simulink model "deva"  (R2015a)
settings: Solver=ode45  StartTime=0.0  StopTime=120  RelTol=1e-3
undefined symbols (not defined in the file): b, m
settings Model: Creator=user  LastModifiedBy=user

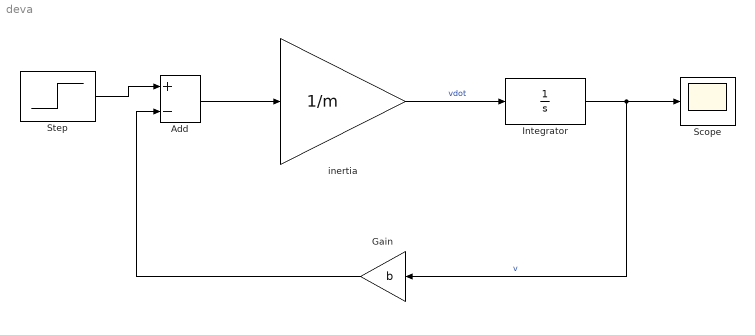
== system deva ==
  Add : Sum  Inputs=+-
  Gain : Gain  Gain=b
  Integrator : Integrator
  Scope : Scope
  Step : Step  Time=0  After=u  SampleTime=0
  inertia : Gain  Gain=1/m
  wires:
  inertia/1 -> Integrator/1  "vdot"
  Integrator/1 -> Gain/1, Scope/1  "v"
  Step/1 -> Add/1
  Add/1 -> inertia/1
  Gain/1 -> Add/2
